simulink model "Vibration_Absorber"  (R2020b)
settings: Solver=VariableStepAuto  StartTime=0.0  StopTime=10  RelTol=1e-3
values from neighbouring files (symbols this model uses):
  b = 50    [data.m]
  k1 = 50    [data.m]
  k2 = 10    [data.m]
  m1 = 100    [data.m]
  m2 = 25    [data.m]
settings Model: Creator=vijay jagtap  LastModifiedBy=vijay jagtap

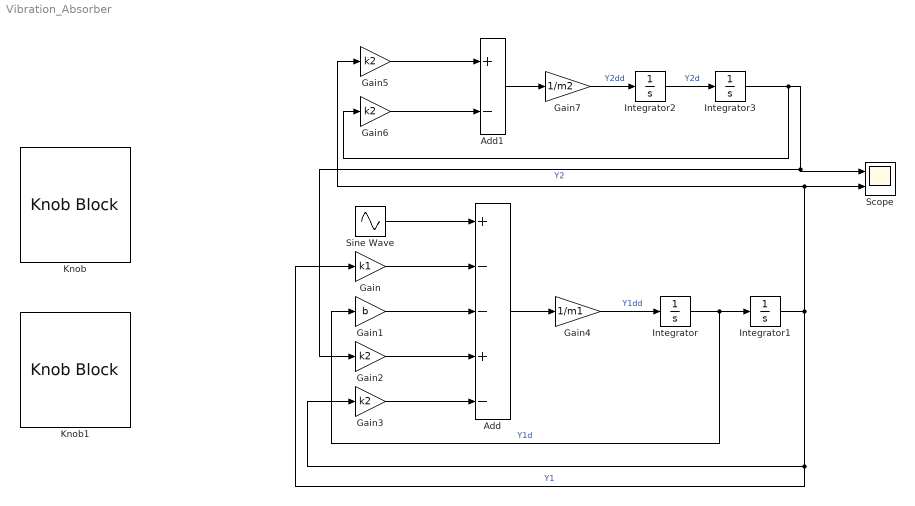
== system Vibration_Absorber ==
  Add : Sum  Inputs=+--+-
  Add1 : Sum  Inputs=+-
  Gain : Gain  Gain=k1
  Gain1 : Gain  Gain=b
  Gain{2..3,5..6} (4 alike) : Gain  Gain=k2
  Gain4 : Gain  Gain=1/m1
  Gain7 : Gain  Gain=1/m2
  Integrator{,1..3} (4 alike) : Integrator
  Knob : KnobBlock  ScaleMax=50
  Knob1 : KnobBlock
  Scope : Scope  NumInputPorts=2
  Sine Wave : Sin  Amplitude=2  Frequency=10  SampleTime=0
  wires:
  Gain3/1 -> Add/5
  Gain2/1 -> Add/4
  Gain1/1 -> Add/3
  Gain/1 -> Add/2
  Add/1 -> Gain4/1
  Gain4/1 -> Integrator/1  "Y1dd"
  Integrator/1 -> Gain1/1, Integrator1/1  "Y1d"
  Integrator1/1 -> Scope/2, Gain5/1, Gain3/1, Gain/1  "Y1"
  Gain6/1 -> Add1/2
  Gain5/1 -> Add1/1
  Add1/1 -> Gain7/1
  Gain7/1 -> Integrator2/1  "Y2dd"
  Integrator2/1 -> Integrator3/1  "Y2d"
  Integrator3/1 -> Gain6/1, Gain2/1, Scope/1  "Y2"
  Sine Wave/1 -> Add/1
